simulink model "vending_MelayModel"  (R2020a)
settings: Solver=FixedStepDiscrete  StartTime=0.0  StopTime=4  FixedStep=0.1  RelTol=1e-3  EnableMultiTasking=on
libraries: simulink x1
settings Model: Creator=The MathWorks, Inc.  LastModifiedBy=INDRAJIT MARATHE
settings DataIOCC: LimitDataPoints=on  SaveFormat=Array  ReturnWorkspaceOutputs=off
settings OptimizationCC: ExpressionDepthLimit=2147483647  InitFltsAndDblsToZero=on  EfficientMapNaN2IntZero=off  LifeSpan=inf
settings DebuggingCC: SaveWithParameterizedLinksMsg=none  UnderspecifiedInitializationDetection=Classic  MergeDetectMultiDrivingBlocksExec=none  SignalResolutionControl=TryResolveAllWithWarning  SolverPrmCheckMsg=warning  MultiTaskDSMMsg=warning  MultiTaskCondExecSysMsg=none  FcnCallInpInsideContextMsg=warning  StateNameClashWarn=warning  SFUnexpectedBacktrackingDiag=warning  SFNoUnconditionalDefaultTransitionDiag=warning  SFExecutionAtInitializationDiag=none  ArithmeticOperatorsInVariantConditions=warning
settings HardwareCC: ProdBitPerPointer=32  ProdBitPerSizeT=32  ProdBitPerPtrDiffT=32  ProdLargestAtomicFloat=None  ProdIntDivRoundTo=Undefined  ProdEndianess=Unspecified  ProdWordSize=32  ProdHWDeviceType=32-bit Generic
settings ModelReferenceCC: PropagateSignalLabelsOutOfModel=off
settings SFSimCC: SimUseLocalCustomCode=off  SimParseCustomCode=off  CustomCodeUndefinedFunction=UseInterfaceOnly
settings RTWCC: RTWUseLocalCustomCode=off
settings CodeAppCC: StateflowObjectComments=on
settings GRTTargetCC: TargetFcnLib=ansi_tfl_tmw.mat  TargetLangStandard=C89/C90 (ANSI)  CombineOutputUpdateFcns=off  GRTInterface=on
settings ConfigComp: CovMetricSettings=dw  CovHtmlReporting=on  CovSaveCumulativeToWorkspaceVar=on  CovSaveSingleToWorkspaceVar=on  CovExternalEMLEnable=off  CovSFcnEnable=off

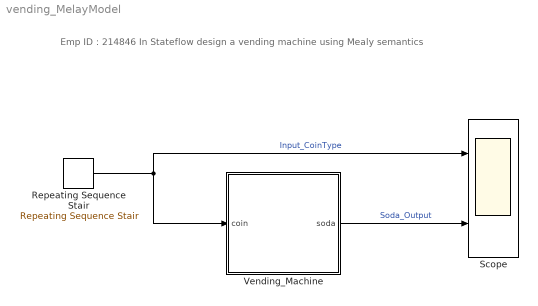
== system vending_MelayModel ==
  note: Emp ID : 214846
      |
      | In Stateflow design a vending machine using Mealy semantics
  " Repeating Sequence Stair" : simulink/Sources/Repeating Sequence Stair  OutValues="[2 1 1 1 1 2  2 1 2 1 2 1 2 ].'"  tsamp=-1  OutMin=[]  OutMax=[]  OutDataTypeStr=double  OutputDataTypeScalingMode=double  OutDataType=fixdt(0,8)  ConRadixGroup=Best Precision: Vector-wise  OutScaling=2^-12
  " Scope" : Scope  NumInputPorts=2
  Vending_Machine : Stateflow chart  TreatAsAtomicUnit=on
  wires:
  Vending_Machine/1(soda) -> " Scope"/2  "Soda_Output"
  " Repeating Sequence Stair"/1 -> " Scope"/1, Vending_Machine/1(coin)  "Input_CoinType"

== stateflow chart vending_MelayModel/Vending_Machine ==
  settings: stateMachineType=MEALY_MACHINE  initializeOutput=1
  state freeState
  state nickel_Inserted
  state dime_Inserted
  (default) -> freeState
  freeState -> nickel_Inserted [order 1] : [coin==1]{soda=0}
  nickel_Inserted -> freeState [order 2] : [coin==2]{soda=1}
  dime_Inserted -> freeState [order 1] : [coin==1]{soda=1}
  freeState -> dime_Inserted [order 2] : [coin==2]{soda=0}
  nickel_Inserted -> dime_Inserted [order 1] : [coin==1]{soda=0}
  dime_Inserted -> nickel_Inserted [order 2] : [coin==2]{soda=1}
  data: coin input double; soda output boolean
